simulink model "Even_Software_rezonator_2_layers_NN_parameterised_tested"  (R2019a)
settings: Solver=VariableStepAuto  StartTime=0.0  StopTime=inf  FixedStep=0.000001  RelTol=1e-3
libraries: simulink x1
settings Model: NumberOfSteps=16  Creator=vardhah  LastModifiedBy=vardhah
settings DataIOCC: ReturnWorkspaceOutputs=off
settings DebuggingCC: UnderSpecifiedDimensionMsg=warning  ArithmeticOperatorsInVariantConditions=warning

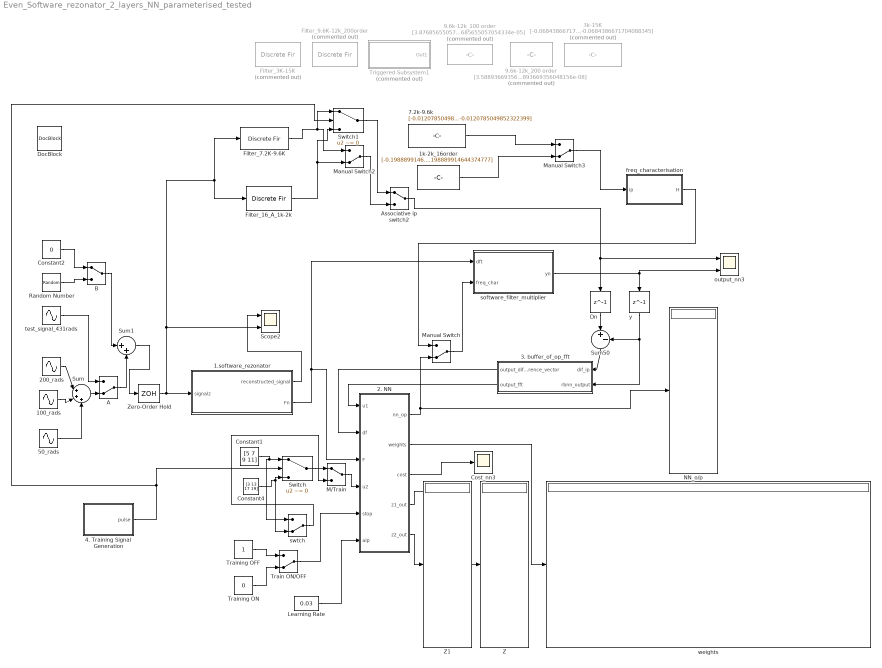
== system Even_Software_rezonator_2_layers_NN_parameterised_tested ==
  " software_filter_multiplier" : MATLAB Function  TreatAsAtomicUnit=on
  1.software_rezonator : MATLAB Function  TreatAsAtomicUnit=on
  100_rads : Sin  Frequency=100  SampleTime=0
  1k-2k_16order : Constant  Value=[-0.198889914644374777 0.0882189428518377339 0.0736891495871065116 0.0638368801789635787 0.0566372642221577294 0.0523172683654103132 0.0494565343907736044 0.048157521822162791 0.048157521822162791 0.0494565343907736044 0.0523172683654103132 0.0566372642221577294 0.0638368801789635787 0.0736891495871065116 0.0882189428518377339 -0.198889914644374777]  VectorParams1D=off
  2. NN : MATLAB Function  TreatAsAtomicUnit=on
  200_rads : Sin  Frequency=200  SampleTime=0
  3. buffer_of_op_fft : MATLAB Function  TreatAsAtomicUnit=on
  3k-15K : Constant  Commented=on  Value=[-0.0684386671704088345 -0.0216035519389094557 -0.0869907772510868094 -0.0695372998678755599 0.0160068430386171648 -0.171506412844009415 -0.104404398490726372 0.48413102780480427 0.48413102780480427 -0.104404398490726372 -0.171506412844009415 0.0160068430386171648 -0.0695372998678755599 -0.0869907772510868094 -0.0216035519389094557 -0.0684386671704088345]  VectorParams1D=off
  4. Training Signal Generation : MATLAB Function  TreatAsAtomicUnit=on
  50_rads : Sin  Frequency=50  SampleTime=0
  "7.2k-9.6k " : Constant  Value=[-0.0120785049852322399 -0.0942455273574688279 0.0101245004695954266 0.125460404555770566 0.034165372769331126 -0.1614987160724079 -0.0984930555982914957 0.150982315564688691 0.150982315564688691 -0.0984930555982914957 -0.1614987160724079 0.034165372769331126 0.125460404555770566 0.0101245004695954266 -0.0942455273574688279 -0.0120785049852322399]  VectorParams1D=off
  9.6k-12k_100 order : Constant  Commented=on  Value=[3.87685655057054334e-05 0.000108803053226908729 -8.26167990877867136e-05 -0.000293336203733274498 2.6285942662608911e-05 0.000470643257144739719 0.000128704829547001234 -0.000409932472117148169 -0.000168878837800233775 5.29388077798551043e-06 -0.000285438581748162664 0.000476496961661710902 0.00138356120682394616 -0.000476433595901257331 -0.00260989841330203781 -0.000263832520003181659 0.00288776740876196033 0.00103696232298899297 -0.00148535664212565491 -0.00029781571721707251 -0.000910294888597508478 -0.00301220003423313329 0.00221471961553778218 0.00782175074594450466 -0.000709211369068674449 -0.0107696105008747954 -0.00258145844866515843 0.00855726436285330835 0.00338081517511367325 -0.00144715698429817813 0.00287506321799563301 -0.00544178445149644165 -0.016125692798747971 0.00552050119563736973 0.0291833518348223603 0.00265487109805798843 -0.0313375380418604021 -0.0109425432817974923 0.0170337904278449956 0.00463136074451602191 0.00673385154025073988 0.0271658069884841494 -0.0215094126752095813 -0.080672987166974186 0.00848125715451410883 0.135328268501058141 0.0372155688614851238 -0.164113227506699488 -0.099857601639362345 0.150463696417151488 0.150463696417151488 -0.099857601639362345 -0.164113227506699488 0.0372155688614851238 0.135328268501058141 0.00848125715451410883 -0.080672987166974186 -0.0215094126752095813 0.0271658069884841494 0.00673385154025073988 0.00463136074451602191 0.0170337904278449956 -0.0109425432817974923 -0.0313375380418604021 0.00265487109805798843 0.0291833518348223603 0.00552050119563736973 -0.016125692798747971 -0.00544178445149644165 0.00287506321799563301 -0.00144715698429817813 0.00338081517511367325 0.00855726436285330835 -0.00258145844866515843 -0.0107696105008747954 -0.000709211369068674449 0.00782175074594450466 0.00221471961553778218 -0.00301220003423313329 -0.000910294888597508478 -0.00029781571721707251 -0.00148535664212565491 0.00103696232298899297 0.00288776740876196033 -0.000263832520003181659 -0.00260989841330203781 -0.000476433595901257331 0.00138356120682394616 0.000476496961661710902 -0.000285438581748162664 5.29388077798551043e-06 -0.000168878837800233775 -0.000409932472117148169 0.000128704829547001234 0.000470643257144739719 2.6285942662608911e-05 -0.000293336203733274498 -8.26167990877867136e-05 0.000108803053226908729 3.87685655057054334e-05]  VectorParams1D=off
  9.6k-12k_200 order : Constant  Commented=on  Value=[3.58893669356048156e-08 -3.82818873463390521e-08 -2.0321720028023873e-07 4.90359188072874186e-08 5.60695246712035587e-07 1.09660540028249228e-07 -9.02554244437910404e-07 -4.11425973326973434e-07 7.02261176603049468e-07 1.84471216608655933e-07 3.26725285155721724e-07 1.85122942566739851e-06 -1.30883758906231066e-06 -6.26130099657902526e-06 3.05461039932901012e-07 1.09009807667638867e-05 3.23497432520277999e-06 -1.08958455239369133e-05 -4.97738604970975483e-06 2.96863479339988865e-06 -4.0832027868080837e-06 8.18297554751245384e-06 2.96530358064679952e-05 -9.55109847507026519e-06 -6.23922165547140565e-05 -7.71216677200245448e-06 7.59750359409520817e-05 2.93209615001356784e-05 -4.65187720652641962e-05 -1.41370609590419019e-05 -1.56985235131491563e-05 -7.53719240448361523e-05 5.59153495137252289e-05 0.000221327384655395267 -1.66050969068338295e-05 -0.000328656395451828759 -8.51260959631819787e-05 0.000282645117406031716 0.000119666235755805559 -6.72511324233616883e-05 7.71213722411986897e-05 -0.000163098688300092245 -0.000529184616157781082 0.000174782969900715956 0.000998932721197958676 0.000103789032707165716 -0.00109406787912954759 -0.000393069844497760581 0.000605548903230077127 0.00017901057135702881 0.000188671213168486616 0.0008317537932211581 -0.000616428076574026661 -0.00225801358273229787 0.000189644939633113819 0.00309786671618311488 0.000749066198738662951 -0.00246959577998202753 -0.000999305917144800888 0.000543345759446133242 -0.000591058888909330575 0.00125474640273121702 0.00385350017895572799 -0.0012819719093164299 -0.00685815514325687284 -0.000643891365732486565 0.00710257598433050412 0.00245016739238454462 -0.00372825461824609263 -0.00107354982596571057 -0.00112558364252808812 -0.00473944354418633605 0.00351472715485449472 0.0123820578712038748 -0.0011101460878915094 -0.0164148510072775998 -0.00382732465676402251 0.0127139357915301426 0.00503981617377440537 -0.00272012803122949386 0.00293385456875478335 -0.00629326791759583608 -0.0189964846306969505 0.00647240842885716226 0.0339172426787937645 0.00302977722420997957 -0.0357411919442247455 -0.0123754194694439944 0.0194465496197908511 0.00571238915438039823 0.00633940801538525594 0.0275121602229752085 -0.0219528139243238031 -0.0822938722183100269 0.00864574898877375209 0.1372509242650502 0.0376134106872798024 -0.165584050427181245 -0.100574100965544921 0.151437569678198519 0.151437569678198519 -0.100574100965544921 -0.165584050427181245 0.0376134106872798024 0.1372509242650502 0.00864574898877375209 -0.0822938722183100269 -0.0219528139243238031 0.0275121602229752085 0.00633940801538525594 0.00571238915438039823 0.0194465496197908511 -0.0123754194694439944 -0.0357411919442247455 0.00302977722420997957 0.0339172426787937645 0.00647240842885716226 -0.0189964846306969505 -0.00629326791759583608 0.00293385456875478335 -0.00272012803122949386 0.00503981617377440537 0.0127139357915301426 -0.00382732465676402251 -0.0164148510072775998 -0.0011101460878915094 0.0123820578712038748 0.00351472715485449472 -0.00473944354418633605 -0.00112558364252808812 -0.00107354982596571057 -0.00372825461824609263 0.00245016739238454462 0.00710257598433050412 -0.000643891365732486565 -0.00685815514325687284 -0.0012819719093164299 0.00385350017895572799 0.00125474640273121702 -0.000591058888909330575 0.000543345759446133242 -0.000999305917144800888 -0.00246959577998202753 0.000749066198738662951 0.00309786671618311488 0.000189644939633113819 -0.00225801358273229787 -0.000616428076574026661 0.0008317537932211581 0.000188671213168486616 0.00017901057135702881 0.000605548903230077127 -0.000393069844497760581 -0.00109406787912954759 0.000103789032707165716 0.000998932721197958676 0.000174782969900715956 -0.000529184616157781082 -0.000163098688300092245 7.71213722411986897e-05 -6.72511324233616883e-05 0.000119666235755805559 0.000282645117406031716 -8.51260959631819787e-05 -0.000328656395451828759 -1.66050969068338295e-05 0.000221327384655395267 5.59153495137252289e-05 -7.53719240448361523e-05 ...(+757 chars)]  VectorParams1D=off
  A : ManualSwitch  CurrentSetting=0
  Associative ip switch2 : ManualSwitch
  "B " : ManualSwitch
  Constant1 : Constant  Value=[5 7 9 11]
  Constant2 : Constant  Value=0
  Constant4 : Constant  Value=[3 13 17 19]
  Cost_nn3 : Scope
  Dn : Delay  DelayLength=1  InitialCondition=0
  DocBlock : simulink/Model-Wide Utilities/DocBlock  DocumentType=Text
      content=|
      | This model consist of complete RBNN for 3 layer NN & scalable number of rezonator.
      | POints to keep in mind while playing with the model.
      |
      | There are various parameter to tune to a list of variable parameter will be helpful.
      |   > Number of rezonators(numberofrezonators).
      |   > Input association signal (size)(u2).
      |   > training batch size (decide u1(input space of feedback) & df(output difference vector)).
      |   > number of layers in NN (layer0=u1+u2 ; layer1 & layer2 => as per user;
      |     Layer3(output layer)= numberofrezonator.
      |   > Output layer must match with number of rezonators.
      |
      | There are 5 major function blocks, that are in use currently. Some need to be configured listed as:
      | 1. software_rezonator
      | 2. NN
      | 3. buffer_of_op_fft
      | 4. Training signal generation
      |
      |
      | Major changes:
      | (a) Number of parallel rezonators
      |     Just change the variable 'numberofrezonator' to required number
      | (b) Input assocaitive signal
      |     1. change the vector input 'constant block'(all associative signal should have same size) 2.change variable 'E' to number of
      |      vectors input.
      |      If deployed in function form, input u2 must be 'column vector'.
      | (c) Training size: change in 2.NN 3.Buffer_of_op_fft 4. Training Signal Generation block
      |     currently it support training size up to 1024, but 8,16 & 32 are recommended size.
      |     Larger the number , greater the time to train.
  Filter_16_A_1k-2k : DiscreteFir  Tag=BlockMethodSubSystem  Coefficients=[-0.198889914644374777 0.0882189428518377339 0.0736891495871065116 0.0638368801789635787 0.0566372642221577294 0.0523172683654103132 0.0494565343907736044 0.048157521822162791 0.048157521822162791 0.0494565343907736044 0.0523172683654103132 0.0566372642221577294 0.0638368801789635787 0.0736891495871065116 0.0882189428518377339 -0.198889914644374777]  InputProcessing=Columns as channels (frame based)
  Filter_3K-15K : DiscreteFir  Tag=BlockMethodSubSystem  Commented=on  Coefficients=[-0.0684386671704088345 -0.0216035519389094557 -0.0869907772510868094 -0.0695372998678755599 0.0160068430386171648 -0.171506412844009415 -0.104404398490726372 0.48413102780480427 0.48413102780480427 -0.104404398490726372 -0.171506412844009415 0.0160068430386171648 -0.0695372998678755599 -0.0869907772510868094 -0.0216035519389094557 -0.0684386671704088345]  InputProcessing=Columns as channels (frame based)
  "Filter_7.2K-9.6K " : DiscreteFir  Tag=BlockMethodSubSystem  Coefficients=[-0.0120785049852322399 -0.0942455273574688279 0.0101245004695954266 0.125460404555770566 0.034165372769331126 -0.1614987160724079 -0.0984930555982914957 0.150982315564688691 0.150982315564688691 -0.0984930555982914957 -0.1614987160724079 0.034165372769331126 0.125460404555770566 0.0101245004695954266 -0.0942455273574688279 -0.0120785049852322399]  InputProcessing=Columns as channels (frame based)
  Filter_9.6K-12k_200order : DiscreteFir  Tag=BlockMethodSubSystem  Commented=on  Coefficients=[3.58893669356048156e-08 -3.82818873463390521e-08 -2.0321720028023873e-07 4.90359188072874186e-08 5.60695246712035587e-07 1.09660540028249228e-07 -9.02554244437910404e-07 -4.11425973326973434e-07 7.02261176603049468e-07 1.84471216608655933e-07 3.26725285155721724e-07 1.85122942566739851e-06 -1.30883758906231066e-06 -6.26130099657902526e-06 3.05461039932901012e-07 1.09009807667638867e-05 3.23497432520277999e-06 -1.08958455239369133e-05 -4.97738604970975483e-06 2.96863479339988865e-06 -4.0832027868080837e-06 8.18297554751245384e-06 2.96530358064679952e-05 -9.55109847507026519e-06 -6.23922165547140565e-05 -7.71216677200245448e-06 7.59750359409520817e-05 2.93209615001356784e-05 -4.65187720652641962e-05 -1.41370609590419019e-05 -1.56985235131491563e-05 -7.53719240448361523e-05 5.59153495137252289e-05 0.000221327384655395267 -1.66050969068338295e-05 -0.000328656395451828759 -8.51260959631819787e-05 0.000282645117406031716 0.000119666235755805559 -6.72511324233616883e-05 7.71213722411986897e-05 -0.000163098688300092245 -0.000529184616157781082 0.000174782969900715956 0.000998932721197958676 0.000103789032707165716 -0.00109406787912954759 -0.000393069844497760581 0.000605548903230077127 0.00017901057135702881 0.000188671213168486616 0.0008317537932211581 -0.000616428076574026661 -0.00225801358273229787 0.000189644939633113819 0.00309786671618311488 0.000749066198738662951 -0.00246959577998202753 -0.000999305917144800888 0.000543345759446133242 -0.000591058888909330575 0.00125474640273121702 0.00385350017895572799 -0.0012819719093164299 -0.00685815514325687284 -0.000643891365732486565 0.00710257598433050412 0.00245016739238454462 -0.00372825461824609263 -0.00107354982596571057 -0.00112558364252808812 -0.00473944354418633605 0.00351472715485449472 0.0123820578712038748 -0.0011101460878915094 -0.0164148510072775998 -0.00382732465676402251 0.0127139357915301426 0.00503981617377440537 -0.00272012803122949386 0.00293385456875478335 -0.00629326791759583608 -0.0189964846306969505 0.00647240842885716226 0.0339172426787937645 0.00302977722420997957 -0.0357411919442247455 -0.0123754194694439944 0.0194465496197908511 0.00571238915438039823 0.00633940801538525594 0.0275121602229752085 -0.0219528139243238031 -0.0822938722183100269 0.00864574898877375209 0.1372509242650502 0.0376134106872798024 -0.165584050427181245 -0.100574100965544921 0.151437569678198519 0.151437569678198519 -0.100574100965544921 -0.165584050427181245 0.0376134106872798024 0.1372509242650502 0.00864574898877375209 -0.0822938722183100269 -0.0219528139243238031 0.0275121602229752085 0.00633940801538525594 0.00571238915438039823 0.0194465496197908511 -0.0123754194694439944 -0.0357411919442247455 0.00302977722420997957 0.0339172426787937645 0.00647240842885716226 -0.0189964846306969505 -0.00629326791759583608 0.00293385456875478335 -0.00272012803122949386 0.00503981617377440537 0.0127139357915301426 -0.00382732465676402251 -0.0164148510072775998 -0.0011101460878915094 0.0123820578712038748 0.00351472715485449472 -0.00473944354418633605 -0.00112558364252808812 -0.00107354982596571057 -0.00372825461824609263 0.00245016739238454462 0.00710257598433050412 -0.000643891365732486565 -0.00685815514325687284 -0.0012819719093164299 0.00385350017895572799 0.00125474640273121702 -0.000591058888909330575 0.000543345759446133242 -0.000999305917144800888 -0.00246959577998202753 0.000749066198738662951 0.00309786671618311488 0.000189644939633113819 -0.00225801358273229787 -0.000616428076574026661 0.0008317537932211581 0.000188671213168486616 0.00017901057135702881 0.000605548903230077127 -0.000393069844497760581 -0.00109406787912954759 0.000103789032707165716 0.000998932721197958676 0.000174782969900715956 -0.000529184616157781082 -0.000163098688300092245 7.71213722411986897e-05 -6.72511324233616883e-05 0.000119666235755805559 0.000282645117406031716 -8.51260959631819787e-05 -0.000328656395451828759 -1.66050969068338295e-05 0.000221327384655395267 5.59153495137252289e-05 -7.53719240448361523e-05 ...(+757 chars)]  InputProcessing=Columns as channels (frame based)
  Learning Rate : Constant  Value=0.03
  "M/Train " : ManualSwitch  varsize=on
  Manual Switch : ManualSwitch  CurrentSetting=0  varsize=on
  Manual Switch2 : ManualSwitch  CurrentSetting=0
  Manual Switch3 : ManualSwitch  CurrentSetting=0
  NN_o/p : Display
  Random Number : RandomNumber  Variance=0.01  SampleTime=0.00001
  Scope2 : Scope  NumInputPorts=2
  Sum : Sum  Inputs=|+++
  Sum1 : Sum  Inputs=|++
  Sum50 : Sum  Inputs=|+-
  Switch : Switch  Criteria=u2 ~= 0
  Switch1 : Switch  Criteria=u2 ~= 0
  Train ON/OFF : ManualSwitch  CurrentSetting=0
  Training OFF : Constant
  Training ON : Constant  Value=0
  Triggered Subsystem1 : Subsystem  Commented=on  TreatAsAtomicUnit=on
  Z : Display
  Z1 : Display
  Zero-Order Hold : ZeroOrderHold  SampleTime=0.0001
  freq_characterisation : MATLAB Function  TreatAsAtomicUnit=on
  output_nn3 : Scope  NumInputPorts=2
  swtch : ManualSwitch  CurrentSetting=0
  test_signal_431rads : Sin  Frequency=431  SampleTime=0
  weights : Display
  y : Delay  DelayLength=1  InitialCondition=0
  wires:
  1.software_rezonator/1(reconstructed_signal) -> Scope2/1
  1.software_rezonator/2(Fn) -> " software_filter_multiplier"/1(dft), 2. NN/3(F)
  " software_filter_multiplier"/1(yn) -> output_nn3/2, y/1
  Zero-Order Hold/1 -> Scope2/2, "Filter_7.2K-9.6K "/1, Filter_16_A_1k-2k/1, 1.software_rezonator/1(signalz)
  200_rads/1 -> Sum/1
  100_rads/1 -> Sum/2
  50_rads/1 -> Sum/3
  Filter_16_A_1k-2k/1 -> Switch1/3, Manual Switch2/2
  Dn/1 -> Sum50/1
  y/1 -> 3. buffer_of_op_fft/2(rbnn_output), Sum50/2
  Manual Switch/1 -> " software_filter_multiplier"/2(freq_char)
  freq_characterisation/1(H) -> Manual Switch/1
  2. NN/1(nn_op) -> Manual Switch/2, NN_o/p/1
  Train ON/OFF/1 -> 2. NN/5(stop)
  Training OFF/1 -> Train ON/OFF/1
  Training ON/1 -> Train ON/OFF/2
  Constant1/1 -> Switch/1, swtch/1
  Constant4/1 -> swtch/2, Switch/3
  2. NN/3(cost) -> Cost_nn3/1
  2. NN/2(weights) -> weights/1
  2. NN/4(z1_out) -> Z/1
  1k-2k_16order/1 -> Manual Switch3/2
  "7.2k-9.6k "/1 -> Manual Switch3/1
  Manual Switch3/1 -> freq_characterisation/1(ip)
  4. Training Signal Generation/1(pulse) -> Switch/2, Switch1/2
  "Filter_7.2K-9.6K "/1 -> Switch1/1, Manual Switch2/1
  Switch/1 -> "M/Train "/1
  "M/Train "/1 -> 2. NN/4(u2)
  swtch/1 -> "M/Train "/2
  Associative ip switch2/1 -> output_nn3/1, Dn/1
  Switch1/1 -> Associative ip switch2/1
  2. NN/5(z2_out) -> Z1/1
  3. buffer_of_op_fft/1(output_difference_vector) -> 2. NN/2(df)
  Sum50/1 -> 3. buffer_of_op_fft/1(dif_ip)
  3. buffer_of_op_fft/2(output_fft) -> 2. NN/1(u1)
  Learning Rate/1 -> 2. NN/6(alp)
  Manual Switch2/1 -> Associative ip switch2/2
  test_signal_431rads/1 -> A/1
  Sum/1 -> A/2
  Sum1/1 -> Zero-Order Hold/1
  A/1 -> Sum1/2
  Constant2/1 -> "B "/1
  Random Number/1 -> "B "/2
  "B "/1 -> Sum1/1

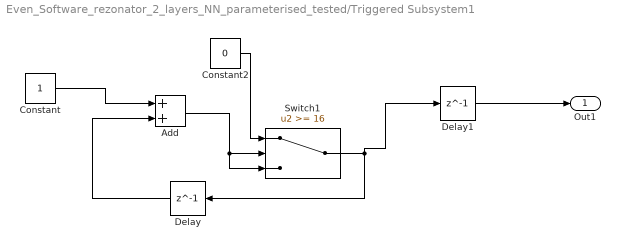
== system Even_Software_rezonator_2_layers_NN_parameterised_tested/Triggered Subsystem1 ==
  Add : Sum
  Constant : Constant
  Constant2 : Constant  Value=0
  Delay : Delay  DelayLength=1  InitialCondition=0
  Delay1 : Delay  DelayLength=1  InitialCondition=0
  Switch1 : Switch  Threshold=16
  Out1 : Outport
  wires:
  Constant2/1 -> Switch1/1
  Constant/1 -> Add/1
  Switch1/1 -> Delay1/1, Delay/1
  Delay/1 -> Add/2
  Add/1 -> Switch1/3, Switch1/2
  Delay1/1 -> Out1/1

== matlab function Even_Software_rezonator_2_layers_NN_parameterised_tested/2. NN ==
  settings: sampleTime=0.01
  data: u1 input; df input; F input; u2 input; nn_op output; weights output; cost output; z1_out output; stop input; z2_out output; alp input
function [nn_op,weights,cost,z1_out,z2_out]  = NN(u1,df,F,u2,stop,alp)

persistent w1 w2;
persistent vy;
persistent g1 g2;
persistent itr;
persistent J;
persistent del_w1 del_w2;
persistent mult1 mult2 ;
persistent memory_alloc_flag;
persistent n;

%%
%%%%%%----------------------------------------------------------------------------%%%%%
%Hyper-parameter & other tunable part of code

M=16;   %declare batch size of training (It will also be equal to number of input in our case as we are using DFT)
E=4;    % size of external associative input

%layer declaration
layer_1=16;
layer_2=16;       % Output layer must match with number of rezonators declared in rezonator function

%learning rate. Currently reading from input pin 
alpha = alp;

%others
input_layer =M+E;       %layer_0
output_layer=layer_2;

% weight Intialisation 
if isempty(w1)
       w1=randn(input_layer,layer_1)*0.1;
end
if isempty(w2)
       w2=randn(layer_1,layer_2)*0.1;
end

%%%%%---------------------------------------------------------------------------------%%%%%

%%

%synchronising clock
if isempty(n)
        n = 0; end
n=n+1;

%%
%Allocation of variables that will be used during runtime( one time execution code) 
if isempty(memory_alloc_flag)
        memory_alloc_flag = 0; 
end
if isempty(mult1)
       mult1=zeros(layer_1,layer_1*input_layer); 
end
if isempty(mult2)
       mult2=zeros(layer_2,layer_1*layer_2); 
end
if isempty(vy)
       vy=zeros(input_layer,M); 
end

if memory_alloc_flag==0
 %write memory allocation for looped code here.It runs once and store it in memory.  
 mult1=[];
 mult2=[];
  for iteration =1:layer_1
   mult1=[mult1;[zeros(1,(iteration-1)*input_layer) ones(1,input_layer) zeros(1,(layer_1-iteration)*input_layer)]];
  end
  for iterate=1:layer_2
   mult2=[mult2;[zeros(1,(iterate-1)*layer_1) ones(1,layer_1) zeros(1,(layer_2-iterate)*layer_1)]];
  end
 
 for k= 1:input_layer
    for j = 1:M 
        if k<=(M/2)+1 && k>=1
            vy(k,j)=(1/M)*cos(pi*(M-j)*(k-1)/(M/2));
        elseif k<=M && k>=(M/2)+1
            vy(k,j)=-(1/M)*sin(pi*(M-j)*(k-1)/(M/2));
        elseif k>M
            vy(k,j)=0;     
        end
    end
 end
 memory_alloc_flag=1; 
end

%%
%============All other Initiaisation =========================>

%Initialisation of delta of weight storage
if isempty(del_w1)
    del_w1=zeros(1,input_layer*layer_1);
end
if isempty(del_w2)
    del_w2=zeros(1,layer_2*layer_1);
end

%Intialising iteration number & cost value. 
if isempty(itr)
    itr=0;
end
if isempty(J)
    J=0;
end


%gradient initialisation(in matrix form)
if isempty(g1)
    g1= zeros(M,input_layer*layer_1);   
end
if isempty(g2)
    g2= zeros(M,layer_1*layer_2);   
end

%%
%Input vector creation code block
x_in = [real(u1(1:(size(u1,2)/2)+1)) imag(u1(1:(size(u1,2)/2)-1))];
v=transpose([x_in transpose(u2)]);

%%
%RBNN core vectorised algorithm implementation 

%--------------->forward propogation ------------>

z1=w1'*v ;
a1=(1./(1+exp(-z1)));
an1=(a1-0.5);
z2=w2'*an1 ;
a2=(1./(1+exp(-z2)));
an2=(a2-0.5);

%-------------> Backward Propogation -------->

%calculation of Nv:
da2_z2=a2.*(1-a2);
dn_a1=w2'.*repmat(da2_z2,1,layer_1);
da1_z1=a1.*(1-a1); 
dn_z1=dn_a1.*repmat(transpose(da1_z1),output_layer,1);
dn_v=dn_z1*w1';   %"This is Nv" 

%calculation of aD, A & B 
aD=transpose(F)*dn_v*vy;
A=[aD;eye(M-1) zeros(M-1,1)];
B=[transpose(F) ; zeros(M-1,size(F,1))]; 

%calculation of Nw(diff of N(v,w) wrt each weights)
dIn_2= da2_z2*transpose(a1);
dn_w2=repmat(dIn_2,1,layer_2).* mult2;

dIn_1= da1_z1*transpose(v);
da1_w1= repmat(dIn_1,1,layer_1).*mult1;
dn_w1=dn_a1*da1_w1;

%gradient updation
g2=A*g2+B*dn_w2;
g1=A*g1+B*dn_w1;

%Training & updation only once in a batch(batch size=M,n=Overall counter) 
if mod(n,M)==0 && stop==0
    del_w1 =alpha*df*1*g1/M ;
    del_w2 =alpha*df*1*g2/M ;
    del_w_reshaped1= reshape(del_w1,[input_layer,layer_1]);
    del_w_reshaped2= reshape(del_w2,[layer_1,layer_2]);
    w1=w1+ del_w_reshaped1;
    w2=w2+ del_w_reshaped2;
    itr=itr+1;
    J= sum(df.^2,'all')/(2*M);
end

%For logging & visulisation purpose
cost=J;
weights=w1;
z1_out=z1;
z2_out=z2;

%NN output assignment
nn_op=an2;


end

== matlab function Even_Software_rezonator_2_layers_NN_parameterised_tested/3. buffer_of_op_fft ==
  data: output_difference_vector output size=[1,1024]; output_fft output size=[1,1024]; dif_ip input; rbnn_output input
function [output_difference_vector,output_fft] = difBuffer(dif_ip,rbnn_output)                      
%%
%Part of code that need to be configured

 sz=16;             % it is size of training batch(get it from NN block)

 %% 
 
%static part of code
 persistent a b;
 if isempty(a)
  a= zeros(1,sz);
 end
 if isempty(b)
  b= zeros(1,sz);
 end
 
  a= circshift(a,1);
  a(1)=dif_ip;
  b= circshift(b,1);
  b(1)=rbnn_output;

 output_difference_vector=a; 
% output_fft=1/sz*fft(b); 
output_fft=b;
 
end

== matlab function Even_Software_rezonator_2_layers_NN_parameterised_tested/freq_characterisation ==
  data: ip input; H output
function H  = freq_character(ip)                      

dft_of_ip=fft(ip); 
size_dft=size(dft_of_ip,2)/2;
H =transpose([real(dft_of_ip(1:size_dft+1)) imag(dft_of_ip(2:size_dft))]);

end

== matlab function Even_Software_rezonator_2_layers_NN_parameterised_tested/1.software_rezonator ==
  data: signalz input; reconstructed_signal output; Fn output size=16
function [reconstructed_signal,Fn]   = rezonator(signalz)

persistent numberofrezonator;
persistent g c bfr_rezo_sm aft_delay dft_out;
persistent out signal_dif;
persistent n;
persistent memory_alloc_flag;


%%
%assign the number of rezonator here. For configuring it for higher order
%rezonator  we need to change (1) 'numberofrezonaotor' variable
if isempty(numberofrezonator)
        numberofrezonator = 16;   %here 16 parallel rezonators
end
%%
%Static Code below
%Initialisation of memory allocations/variables ====> 
if isempty(memory_alloc_flag)
        memory_alloc_flag = 0; 
end
if isempty(g)
       g=zeros(numberofrezonator,numberofrezonator,'like',0i); 
end
if isempty(c)
       c=zeros(numberofrezonator,numberofrezonator,'like',0i); 
end
if memory_alloc_flag==0
 for i=0:numberofrezonator-1
  for j= 0:numberofrezonator-1
   g(i+1,j+1)=1/numberofrezonator*(exp(-1i*2*pi*i*j/numberofrezonator));
   c(i+1,j+1)=(exp(1i*2*pi*i*j/numberofrezonator));
  end 
 end
 memory_alloc_flag=1;
end


%Initialisation of variables  =====> 
if isempty(n)
        n = 0;   
end 
if isempty(out)
  out=0+0i;
end
if isempty(signal_dif)
  signal_dif=0+0i;
end
if isempty(bfr_rezo_sm)
  bfr_rezo_sm=repmat(0+0i,numberofrezonator,1);
end
if isempty(aft_delay)
  aft_delay=repmat(0+0i,numberofrezonator,1);
end
if isempty(dft_out)
  dft_out=repmat(0+0i,numberofrezonator,1);
end

%creating cycle of rotation for selection of correct column of g & c.
cycle=mod(n,numberofrezonator);

%resonator core -----------------------------> 
dft_out=c(:,cycle+1).*aft_delay;
out= sum(dft_out,1);
signal_dif=signalz-out;
bfr_rezo_sm=g(:,cycle+1).*signal_dif;

%counting the counter
n=n+1;

% output assignment ------------------>
reconstructed_signal=out;
dft=aft_delay; 
N=size(dft,1);
a=1:1:N/2-1;
b=N/2+1:1:N-1;
dft_trans=transpose(dft);
Fn=transpose([real(dft_trans(1)) 2*(real(dft_trans(2:N/2)).*cos(2*pi*a*n/N)-imag(dft_trans(2:N/2)).*sin(2*pi*a*n/N)) -1^n*real(dft_trans(N/2+1)) -2*(imag(dft_trans(N/2+2:N)).*cos(2*pi*b*n/N)+real(dft_trans(N/2+2:N)).*sin(2*pi*b*n/N))]);
%--------output assignment over----------<

%final updation of buffer ------>>>>>>>>>>>>
aft_delay= aft_delay+bfr_rezo_sm; 
end

== matlab function Even_Software_rezonator_2_layers_NN_parameterised_tested/ software_filter_multiplier ==
  data: dft input; yn output; freq_char input
function yn = fcn(dft,freq_char)
yn=transpose(freq_char)*dft;
end

== matlab function Even_Software_rezonator_2_layers_NN_parameterised_tested/4. Training Signal Generation ==
  data: pulse output
function pulse   = fcn()
M=16;

persistent cnt;
persistent n;
if isempty(cnt)
    cnt=0;
end
if isempty(n)
    n=0;
end
n=n+1;
if mod(n,M)==0
     cnt=cnt+1;
 end
 pulse = mod(cnt,2);

end
